simulink model "KitGewerk2_v14"  (R2014a)
settings: Solver=ode3  StartTime=0.0  StopTime=inf  FixedStep=0.005  RelTol=1e-3
undefined symbols (not defined in the file): Com1, Com2, none
libraries: slrtlib x14, dspswit3 x3, simulink x2, xpcseriallib x2
(part 2 of 2)

== matlab function KitGewerk2_v14/Robotino/serial communication/error filter & protocol disassembler ==
  settings: sampleTime=dtpc/2
  data: response input; error_free_resp_in input; direction_motor0_out output; velocity_motor0_out output; direction_motor1_out output; velocity_motor1_out output; direction_motor2_out output; velocity_motor2_out output; distance_measuring_sensors_out output; di03_bump_out output; bumper_out output; error_free_resp_out output
%%%%%%%%%%%%%%%%%%%%%%%%%%%%%%%%%%%%%%%%%%%%%%%%%%%%%%%%%%%%%%%%%%%%%%%%%%%
% Error check of the 'I/O-Board to PC104 message' and filtering of this   %
% defective response: Substitute defective message by the last error free %
% message.                                                                %
% Saving of the rotating direction, velocity, shaft position and running  %
% time of the three motors. Combining all shaft positions in a vector.    %
% Combining all running times in a vector.                                %
% Saving of the three bumper bytes indicating a collision in a vector.    %
% Saving the values of the nine distance measuring IR-sensors in a vector.%
%                                                                         %
% inputs: response (actual 'I/O-Board to PC104 message')(vector 102       %
%                   elements)                                             %
%         error_free_resp_in (last error free 'I/O-Board to PC104         %
%                             message')                                   %
% outputs: directions and velocities of the three motors                  %
%          motor_positions_out (shaft positions of the three motors)      %
%                              (vector 12 elements)                       %
%          time_bytes_out (running times of the three motors)             %
%                         (vector 9 elements)                             %
%          distance_measuring_sensors_out (values of the nine IR-sensors) %
%                                         (vector 9 elements)             %
%          bumper_out (vector 3 elements)                                 %
%          error_free_resp_out (error free 'I/O-Board to PC104 message')  %
%                              (vector 102 elements)                      %
%%%%%%%%%%%%%%%%%%%%%%%%%%%%%%%%%%%%%%%%%%%%%%%%%%%%%%%%%%%%%%%%%%%%%%%%%%%
function [direction_motor0_out, velocity_motor0_out, ...
          direction_motor1_out, velocity_motor1_out, ...
          direction_motor2_out, velocity_motor2_out, ...
          distance_measuring_sensors_out, di03_bump_out, bumper_out, ...
          error_free_resp_out] = fcn(response, error_free_resp_in)
%           motor_positions_out, time_bytes_out, ...)
      
%%%%%%%%%%%%%%%%%%%%%%%%%%%%%%%%%%%%%%%%%%%%%%%%%%%%%
% filtering defective 'I/O-Board to PC104 messages' %
%%%%%%%%%%%%%%%%%%%%%%%%%%%%%%%%%%%%%%%%%%%%%%%%%%%%%
if (response(1) == 101) && (response(2) == 82) && (response(3) == 69) ...
   && (response(4) == 67) && (response(100) == 114) ...        % if the ...
   && (response(101) == 101) && (response(102) == 99)  % counter (101), ...
                        % the start (REC) and stop (rec) bytes are true ...
    error_free_resp_out = response;     % save the actual 'I/O-Board to ...
                                                           % PC104 message'
else                                                        % otherwise ...
    error_free_resp_out = error_free_resp_in;     % save the last error ...
                                        % free 'I/O-Board to PC104 message'
end

%%%%%%%%%%%%%%%%%%%%%%%%%%%%%%%%%%%%%%%%%%%%%%%%%%%%%%%%%%%%%%%%%%%%%%%%%%
% save rotating direction, velocity, shaft position and the running time %
% of motor0                                                              %
%%%%%%%%%%%%%%%%%%%%%%%%%%%%%%%%%%%%%%%%%%%%%%%%%%%%%%%%%%%%%%%%%%%%%%%%%%
direction_motor0_out  = error_free_resp_out(26);
velocity_motor0_out   = error_free_resp_out(27);
% position_motor0_byte1 = error_free_resp_out(28);
% position_motor0_byte2 = error_free_resp_out(29);
% position_motor0_byte3 = error_free_resp_out(30);
% position_motor0_byte4 = error_free_resp_out(31);
% time_motor0_byte1     = error_free_resp_out(34);
% time_motor0_byte2     = error_free_resp_out(35);
% time_motor0_byte3     = error_free_resp_out(36);

%%%%%%%%%%%%%%%%%%%%%%%%%%%%%%%%%%%%%%%%%%%%%%%%%%%%%%%%%%%%%%%%%%%%%%%%%%
% save rotating direction, velocity, shaft position and the running time %
% of motor1                                                              %
%%%%%%%%%%%%%%%%%%%%%%%%%%%%%%%%%%%%%%%%%%%%%%%%%%%%%%%%%%%%%%%%%%%%%%%%%%
direction_motor1_out  = error_free_resp_out(47);
velocity_motor1_out   = error_free_resp_out(48);
% position_motor1_byte1 = error_free_resp_out(49);
% position_motor1_byte2 = error_free_resp_out(50);
% position_motor1_byte3 = error_free_resp_out(51);
% position_motor1_byte4 = error_free_resp_out(52);
% time_motor1_byte1     = error_free_resp_out(55);
% time_motor1_byte2     = error_free_resp_out(56);
% time_motor1_byte3     = error_free_resp_out(57);

%%%%%%%%%%%%%%%%%%%%%%%%%%%%%%%%%%%%%%%%%%%%%%%%%%%%%%%%%%%%%%%%%%%%%%%%%%
% save rotating direction, velocity, shaft position and the running time %
% of motor2                                                              %
%%%%%%%%%%%%%%%%%%%%%%%%%%%%%%%%%%%%%%%%%%%%%%%%%%%%%%%%%%%%%%%%%%%%%%%%%%
direction_motor2_out  = error_free_resp_out(68);
velocity_motor2_out   = error_free_resp_out(69);
% position_motor2_byte1 = error_free_resp_out(70);
% position_motor2_byte2 = error_free_resp_out(71);
% position_motor2_byte3 = error_free_resp_out(72);
% position_motor2_byte4 = error_free_resp_out(73);
% time_motor2_byte1     = error_free_resp_out(76);
% time_motor2_byte2     = error_free_resp_out(77);
% time_motor2_byte3     = error_free_resp_out(78);

%%%%%%%%%%%%%%%%%%%%%%%%%%%%%%%%%%%%%%%%%%%
% save the three bumper bytes in a vector %
%%%%%%%%%%%%%%%%%%%%%%%%%%%%%%%%%%%%%%%%%%%
bumper_out = [error_free_resp_out(32), error_free_resp_out(53), ...
              error_free_resp_out(74)]';
          
%%%%%%%%%%%%%%%%%%%%%%%%%%%%%%%%%%%%%%%%%%%%%%%%%%%%%%%%%%%%%%%%%%%%%%
% save the values of the nine distance measuring sensors in a vector %
%%%%%%%%%%%%%%%%%%%%%%%%%%%%%%%%%%%%%%%%%%%%%%%%%%%%%%%%%%%%%%%%%%%%%%
distance_measuring_sensors_out = [error_free_resp_out(60), ...
                    error_free_resp_out(59), error_free_resp_out(44), ...
                    error_free_resp_out(39), error_free_resp_out(38), ...
                    error_free_resp_out(17), error_free_resp_out(18), ...
                    error_free_resp_out(23), error_free_resp_out(65)];
                
%%%%%%%%%%%%%%%%%%%%%%%%%%%%%%%%%%%%%%%%%%%%%%%%%%%%%%%%
% save positions of the three motor shafts in a vector %
%%%%%%%%%%%%%%%%%%%%%%%%%%%%%%%%%%%%%%%%%%%%%%%%%%%%%%%%
% motor_positions_out = [position_motor0_byte1, position_motor0_byte2, ...
%                        position_motor0_byte3, position_motor0_byte4, ...
%                        position_motor1_byte1, position_motor1_byte2, ...
%                        position_motor1_byte3, position_motor1_byte4, ...
%                        position_motor2_byte1, position_motor2_byte2, ...
%                        position_motor2_byte3, position_motor2_byte4];

%%%%%%%%%%%%%%%%%%%%%%%%%%%%%%%%%%%%%%%%%%%%%%%%%%%%%%%%%%
% save the running times of the three motors in a vector %
%%%%%%%%%%%%%%%%%%%%%%%%%%%%%%%%%%%%%%%%%%%%%%%%%%%%%%%%%%
% time_bytes_out = [time_motor0_byte1, time_motor0_byte2, ...
%                   time_motor0_byte3, time_motor1_byte1, ...
%                   time_motor1_byte2, time_motor1_byte3, ...
%                   time_motor2_byte1, time_motor2_byte2, time_motor2_byte3];

%%%%%%%%%%%%%%%%%%%%%%%%%%%%%%%%%%%%%%
% save values of digital input 0 - 3 %
%%%%%%%%%%%%%%%%%%%%%%%%%%%%%%%%%%%%%%
di03_bump_out = error_free_resp_out(32);

== matlab function KitGewerk2_v14/Robotino/receive direction, unit & velocity converter ==
  settings: sampleTime=dtpc/2
  data: direction_motor0_in input; v_x_out output; velocity_motor0_in input; direction_motor1_in input; velocity_motor1_in input; direction_motor2_in input; velocity_motor2_in input; v_y_out output; v_theta_out output
%%%%%%%%%%%%%%%%%%%%%%%%%%%%%%%%%%%%%%%%%%%%%%%%%%%%%%%%%%%%%%%%%%%%%%%%%%%
% assembly of the three separate positive motor velocities (resolution:   %
% 1Byte) and their rotation direction to positive and/or negative         %
% longitudinal, lateral & rotational velocities (in milimeters per        %
% second)                                                                 %
%                                                                         %
% inputs:  direction_motor0_in (rotating direction of motor0              %
%          (129 := counter-clockwise; 128 := clockwise)),                 %
%          velocity_motor0_in (from 0 to 255),                            %
%          direction_motor1_in (rotating direction of motor1              %
%          (0 := counter-clockwise; 1 := clockwise)),                     %
%          velocity_motor1_in (from 0 to 255),                            %
%          direction_motor2_in (rotating direction of motor2              %
%          (0 := counter-clockwise; 1 := clockwise)),                     %
%          velocity_motor2_in (from 0 to 255)                             %
% outputs: v_x_out (longitudinal velocity (in milimeters per second)),    %
%          v_y_out (lateral velocity (in milimeters per second)),         %
%          v_theta_out (rotational velocity (in milimeters per second))   %
%%%%%%%%%%%%%%%%%%%%%%%%%%%%%%%%%%%%%%%%%%%%%%%%%%%%%%%%%%%%%%%%%%%%%%%%%%%
function [v_x_out, v_y_out, v_theta_out] ...
    = fcn(direction_motor0_in, velocity_motor0_in, direction_motor1_in, ...
          velocity_motor1_in, direction_motor2_in, velocity_motor2_in)
%%%%%%%%%%%%%%%%%%%%%%%%%%%%%%%%%%%%%%%%%%%%%%%%%%%%%%%%%%%%%%%%%
% assembly of absolute motor velocity and rotating direction to %
% longitudinal, lateral & rotational velocity for every motor   %
%%%%%%%%%%%%%%%%%%%%%%%%%%%%%%%%%%%%%%%%%%%%%%%%%%%%%%%%%%%%%%%%%
if direction_motor0_in < 129
    v0 = -velocity_motor0_in;
else
    v0 =  velocity_motor0_in;
end

if direction_motor1_in < 1
    v1 = -velocity_motor1_in;
else
    v1 =  velocity_motor1_in;
end

if direction_motor2_in < 1
    v2 = -velocity_motor2_in;
else
    v2 =  velocity_motor2_in;
end

%%%%%%%%%%%%%%%%%%%%%%%%%%%%%%%%%%%%%%%%%%%%%%%%%%%%%%%%%%%%%%%%%%%%%%%%%
% conversion of the separate motor velocities from a value between -255 %
% and 255 to millimeters                                                %
%%%%%%%%%%%%%%%%%%%%%%%%%%%%%%%%%%%%%%%%%%%%%%%%%%%%%%%%%%%%%%%%%%%%%%%%%
f_rcv = 7.02;
v0    = v0 * f_rcv;
v1    = v1 * f_rcv;
v2    = v2 * f_rcv;

%%%%%%%%%%%%%%%%%%%%%%%%%%%%%%%%%%%%%%%%%%%%%%%%%%%%%%%%%%%%%%%%%%%%
% conversion from three separate motor velocities to longitudinal, %
% lateral & rotational velocity                                    %
%%%%%%%%%%%%%%%%%%%%%%%%%%%%%%%%%%%%%%%%%%%%%%%%%%%%%%%%%%%%%%%%%%%%
v_x_out     = (v2 - v0) / (2 * cosd(30));                         % in mm/s
v_y_out     = (v0 - 2 * v1 + v2) / 3;                             % in mm/s
v_theta_out = (v0 + v1 + v2) / (3 * 135);                        % in rad/s

== matlab function KitGewerk2_v14/Begrenzung ==
  data: win input; wout output
function wout = fnc(win)
wert= zeros(1);
if win > 500
    wert = 500;
else
    wert = win;
end
wout = wert;

== matlab function KitGewerk2_v14/Robotino/serial communication/stop by bumper ==
  settings: sampleTime=2*dtpc
  data: stop_out output; bumper input; stop_flag_in input; stop_flag_out output
%%%%%%%%%%%%%%%%%%%%%%%%%%%%%%%%%%%%%%%%%%%%%%%%%%%%%%%%%%%%%%%%%%%%%%%%%%%
% Recognition of collisions and creating of variables indicating and      %
% marking a collision                                                     %
%                                                                         %
% inputs: bumper (vector of the three bumper bytes)                       %
%         stop_flag_in (As long as no collision has occured,              %
%                       'stop_flag_in' contains the last bumper vector    %
%                       indicating no collision.                          %
%                       If a collision has occured, 'stop_flag_in'        %
%                       contains the last bumper vector indicating a      %
%                       collision until the simulation stops.)            %
% outputs: stop_out (indicates a collision: 1 = no collision;             %
%                                           0 = collision)                %
%          stop_flag_out (gets the actual bumper vector unless 'bumper'   %
%                         indicates no collision and 'stop_flag_in'       %
%                         indicates a past collision.)                    %
%%%%%%%%%%%%%%%%%%%%%%%%%%%%%%%%%%%%%%%%%%%%%%%%%%%%%%%%%%%%%%%%%%%%%%%%%%%
function [stop_out, stop_flag_out] = fcn(bumper, stop_flag_in)
if max(bumper) == 31       % as soon as the maximum value of the bumper ...
                              % vector indicates 31 a collision is detected
    stop_out = 0;
    stop_flag_out = bumper;
elseif max(stop_flag_in) == 31 % if the maximum value of 'stop_flag_in' ...
                                      % indicates a past collision (31) ...
    stop_out = 0;         % 'stop_out' gets 0 for a further stop of the ...
                                                           % motors and ...
    stop_flag_out = stop_flag_in; % 'stop_flag_out' gets the last bumper...
                                       % vector indicating a past collision
else                                                        % otherwise ...
    stop_out = 1;    % 'stop_out' gets 1 to keep the motors running and ...
    stop_flag_out = bumper; % 'stop_flag_out' gets the actual bumper vector
end

== matlab function KitGewerk2_v14/Robotino/distance converter ==
  settings: sampleTime=dtpc/2
  data: dms_in input; dms_out output
%%%%%%%%%%%%%%%%%%%%%%%%%%%%%%%%%%%%%%%%%%%%%%%%%%%%%%%%%%%%%%%%%%%%%%%%%%%
% conversion of the nine distance measuring sensor values (resolution:    %
% 1Byte) to unit milimeters (range: from 40mm to 1500mm) with linear      %
% interpolation                                                           %
%                                                                         %
% input:  vector containing the values of the nine distance measuring     %
%         sensors                                                         %
% output: vector containing the nine values in milimeters                 %
%%%%%%%%%%%%%%%%%%%%%%%%%%%%%%%%%%%%%%%%%%%%%%%%%%%%%%%%%%%%%%%%%%%%%%%%%%%
function dms_out = fcn(dms_in)

y_mm = [40, 45, 50, 60, 75, 100, 125, 150, 175, 200, 250, 300]; % , ...
        %400, 500, 600, 700, 800, 900, 1000, 1100, 1200, 1300, 1500];
    
x_sensor = [255, 249.7733813, 228.6082474, 193.6871795, ...
            152.0044843, 113.7266187, 92.42268041, ...
            76.36407767, 65.19289827, 55.1025641, ...
            43.06299213, 34.97068404]; % , 24.37410072, ...
            % 16.3381295, 11.62589928, 8.661870504, ...
            % 6.316546763, 4.74, 3.65, 2.96, 2.40, ...
            % 2.035971223, 1.539568345];

% x_sensor = round(100 * x_sensor) / 100;

dms_out = interp1(x_sensor, y_mm, dms_in, 'linear');

== matlab function KitGewerk2_v14/Robotino/assemble robotino response ==
  data: v_x_in input; robotino_response output; v_y_in input; v_theta_in input; distance_measuring_sensors_in input; bumper_in input; light_barrier_in input; slider_in input
%%%%%%%%%%%%%%%%%%%%%%%%%%%%%%%%%%%%%%%%%%%%%%%%%%%%%%%%%%%%%%%%%%%%%%%%%%%
% Assembly of robot data in a vector of 34 elements.                      %
%                                                                         %
% inputs:   longitudinal, lateral and rotational velocity (in mm/s),      %
%           shaft positions of the three motors (4 elements per motor),   %
%           running times of the three motors (3 elements per motor),     %
%           values of the nine IR-sensors (in mm),                        %
%           bumper collision (1 = no collision;                           %
%                             0 = collision)                              %
% outputs:  vector containing assembled input data                        %
%%%%%%%%%%%%%%%%%%%%%%%%%%%%%%%%%%%%%%%%%%%%%%%%%%%%%%%%%%%%%%%%%%%%%%%%%%%
function robotino_response = fcn(v_x_in, v_y_in, v_theta_in, ...
                                 distance_measuring_sensors_in, ...
                                 bumper_in, light_barrier_in, slider_in)
                                 % motor_positions_in, time_bytes_in, ...)
robotino_response = [light_barrier_in, slider_in, v_x_in, v_y_in, ...
                     v_theta_in, ...%motor_positions_in, time_bytes_in, ...
                     distance_measuring_sensors_in, bumper_in]';

== matlab function KitGewerk2_v14/Robotino/light barrier & slider ==
  data: di03_bump_in input; light_barrier output; slider output
function [light_barrier, slider] = fcn(di03_bump_in)
%%%%%%%%%%%%%%%%%%%%%%%%%%%%%%%%%%%%%%%%%%%%%%%%%%%%%%%%%%%%%%%%%%%%%%%%%%%
% di03_bump_in = 0 alternatively 12 ->  no light barrier activation       %
%                                       no slider activation              %
% di03_bump_in = 13                 ->  only light barrier activation     %
% di03_bump_in = 14                 ->  only slider activation            %
% di03_bump_in = 15                 ->  light barrier activation          %
%                                       slider activation                 %
%%%%%%%%%%%%%%%%%%%%%%%%%%%%%%%%%%%%%%%%%%%%%%%%%%%%%%%%%%%%%%%%%%%%%%%%%%%
% function [light_barrier, slider] = fcn(di03_bump_in)
% bin = dec2bin(di03_bump_in);
% if bin(3) == 1
%     light_barrier = 1;
% else
%     light_barrier = 0;
% end
% if bin(4) == 1
%     slider = 1;
% else
%     slider = 0;
% end
if     di03_bump_in == 13
    light_barrier = 1;
    slider        = 0;
elseif di03_bump_in == 14
    light_barrier = 0;
    slider        = 1;
elseif di03_bump_in == 15
    light_barrier = 1;
    slider        = 1;
else
    light_barrier = 0;
    slider        = 0;
end

== matlab function KitGewerk2_v14/Begrenzung1 ==
  data: win input; wout output
function wout = fnc(win)
wert= zeros(1);
if win > 500
    wert = 500;
else
    wert = win;
end
wout = wert;

== matlab function KitGewerk2_v14/Begrenzung2 ==
  data: win input; wout output
function wout = fnc(win)
wert= zeros(1);
if win > 3,14
    wert = 3,14;
else
    wert = win;
end
wout = wert;

== matlab function KitGewerk2_v14/Gewerk_2/Kollisionserkennung ==
  data: d_Abstand input; b_stop output boolean; ad_Abstandssensor input
function b_stop = fcn(d_Abstand,ad_Abstandssensor)
b_stop=false;
if sum(isnan(ad_Abstandssensor))==9 % nan = kein Hinderniss
    % kein Hinderniss   
    b_stop= false; 
else
    % Hinderniss entdeckt, min. ein Sensor(kein nan)
    if ( (ad_Abstandssensor(1)<d_Abstand) || (ad_Abstandssensor(2)<d_Abstand) || (ad_Abstandssensor(3)<d_Abstand) || ...
         (ad_Abstandssensor(4)<d_Abstand) ||(ad_Abstandssensor(5)<d_Abstand) ||(ad_Abstandssensor(6)<d_Abstand) || ...
         (ad_Abstandssensor(7)<d_Abstand) || (ad_Abstandssensor(8)<d_Abstand) ||(ad_Abstandssensor(9)<d_Abstand)) 

    b_stop= true;
    end
end

== matlab function KitGewerk2_v14/Gewerk_2/MATLAB Function ==
  data: ad_PL input; d_Y_soll output double; d_X_soll output double; d_Phi_soll output double; d_V_Max_soll output double; int_I input
function [d_Y_soll,d_X_soll,d_Phi_soll,d_V_Max_soll]= fcn(ad_PL,int_I)

int_I=int_I+1; %Offset, da Zeilenindex bei 1 beginnt



if (ad_PL(int_I,1)<0 || ad_PL(int_I,2)<0 || ad_PL(int_I,3)<0 || ad_PL(int_I,4)<0)
int_I = int_I-1;
end 

d_Y_soll= ad_PL(int_I,1);
d_X_soll= ad_PL(int_I,2);
d_Phi_soll= ad_PL(int_I,3);
d_V_Max_soll= ad_PL(int_I,4);

== stateflow chart KitGewerk2_v14/Gewerk_2/Chart ==
  state Routinen_Stationen
    state Wegpunktliste_erstellen_state
      entry: A_WPL=Wegpunktliste_erstellen(UI_Auftrnr,uint8(B_Endst))
      B_WPL_cnt_reset =true
    state Werkstueck_aufnehmen
      state Fahrt_zu_Platz1
        entry: B_WPL_cnt_reset=false
      state Greifer_schließen
        entry:B_WP_weiter=true
        B_Greifer= true
        B_Stop=true
        exit:B_Stop=false
      state Weiterfahren_zu_RFID
        entry:B_WP_weiter=false
      state RFID_lesen_2
        during: UI_to_GW1= uint8(2)
        B_Stop=true
        exit:B_Stop=false
        B_WP_weiter=true
      state WP_weiterschalten_3
      state Routine_fertig
        entry: B_Endst=true
      Fahrt_zu_Platz1 -> Greifer_schließen : [B_Schieber&&B_Lichtschranke]
      Greifer_schließen -> Weiterfahren_zu_RFID : after(500,msec)
      Weiterfahren_zu_RFID -> RFID_lesen_2 : [B_Schieber]
      RFID_lesen_2 -> WP_weiterschalten_3 : [UI_from_GW1==2]
      WP_weiterschalten_3 -> Routine_fertig : /{B_WP_weiter=false}
    state Werkstueck_ablegen
      state Fahrt_zu_RFID
        entry: B_WPL_cnt_reset=false
      state RFID_lesen
        entry: UI_to_GW1= uint8(4)
        B_Stop=true
        exit:B_Stop=false
        B_WP_weiter=true
      state WP_weiterschalten
      state Fahrt_zu_Ablage
        entry: B_WP_weiter=false
      state Greifer_Oeffnen
        entry: B_Stop=true
        B_Greifer=false
        B_WP_weiter=true
      state WP_weiterschalten2
        entry:
        B_Stop=false
      state Auftrag_fertig
        entry: B_WP_weiter=false
        exit:UI_to_GW1= uint8(5)
        B_Endst=false
      Fahrt_zu_RFID -> RFID_lesen : [B_Schieber]
      RFID_lesen -> WP_weiterschalten : [UI_from_GW1==4]
      WP_weiterschalten -> Fahrt_zu_Ablage
      Fahrt_zu_Ablage -> Greifer_Oeffnen : [B_Schieber]
      Greifer_Oeffnen -> WP_weiterschalten2 : after(500,msec)
      WP_weiterschalten2 -> Auftrag_fertig
    (default) -> Wegpunktliste_erstellen_state
    Wegpunktliste_erstellen_state -> Fahrt_zu_RFID [order 1] : [B_Endst==true]
    Wegpunktliste_erstellen_state -> Fahrt_zu_Platz1 [order 2] : [B_Endst==false]
  state Station_aendern
    entry: if B_Endst==false
    UI_Auftrnr=UI_Startstation
    else
    UI_Auftrnr=UI_Endstation
    end
  state Fahrt_in_nav_2
  state Nav2_abfrage
  state Eintrittspunkt_erreicht
  state A_stern_fahrt
    state A_stern
    state Kollisionserkennung
      entry:
      if B_Endst==false
      UI_to_GW1=uint8(1) %Startplatz für GW1 freigeben
      else
      UI_to_GW1=uint8(3) %Endplatz für GW1 freigeben
      end
    A_stern -> Kollisionserkennung : [WP_cnt>1]
        | % Sobald der Zähler>1
        | % befindet sich der
        | % Robi im Feld
    (default) -> A_stern
  state Stationsentscheider
    entry: if B_Endst==false
    UI_Auftrnr=UI_Startstation
    else
    UI_Auftrnr=UI_Endstation
    end
  state Fahrt_zum_Warteplatz
    entry:A_stern_test=simfcn()
    state Out1 = simfcn [function]
  state Auftrag_empfangen
    exit:
    UI_Startstation=UI_Startstation_in
    UI_Endstation=UI_Endstation_in
    %Eingänge speichern
  state Init
    entry: B_Endst=false
  state Warten_auf_Auftrag
  state Warten_auf_neuen_Auftrag
  state Routinen_Warteplaetze
  state Routinen_Ladestationen
    state Warten_auf_Ereignis
    state Laden_beenden
    state Laden_beginnen
    state Fahrt_an_rand_nav1
    state Wegpunkte
    state Kontakt_fehler
    Laden_beenden -> Fahrt_an_rand_nav1
    Wegpunkte -> Laden_beginnen : [B_last_WP && B_da]
    Laden_beginnen -> Warten_auf_Ereignis [order 2]
    (default) -> Wegpunkte
    Warten_auf_Ereignis -> Laden_beenden
    Kontakt_fehler -> Laden_beginnen : [B_last_WP && B_da]
    Laden_beginnen -> Kontakt_fehler [order 1]
  state Auftrag_empfangen1
    exit:
    UI_Startstation=UI_Startstation_in
    UI_Endstation=UI_Endstation_in
    %Eingänge speichern
  Kollisionserkennung -> Eintrittspunkt_erreicht : [B_last_WP && B_da ...
      | &&( UI_from_GW1==1 || UI_from_GW1==3)]
  Nav2_abfrage -> A_stern_fahrt [order 1]
  Fahrt_an_rand_nav1 -> Stationsentscheider : [B_last_WP && B_da]
  Station_aendern -> Routinen_Stationen
  Fahrt_in_nav_2 -> Station_aendern
  Eintrittspunkt_erreicht -> Routinen_Stationen [order 1] : [UI_Auftrnr<=16]
  Nav2_abfrage -> Fahrt_in_nav_2 [order 2]
  Warten_auf_Auftrag -> Auftrag_empfangen : [UI_Startstation_in==200 ...
      | && UI_Endstation_in==200]...
      |  /{UI_to_GW1= uint8(200)}
  Auftrag_empfangen -> Stationsentscheider : [UI_Startstation_in<200 ...
      | && UI_Endstation_in<200]
  Fahrt_zum_Warteplatz -> Warten_auf_Auftrag : [B_last_WP && B_da]
  Init -> Fahrt_zum_Warteplatz
  Eintrittspunkt_erreicht -> Routinen_Warteplaetze [order 2] : [UI_Auftrnr>16 &&  UI_Auftrnr<=20]
  Stationsentscheider -> A_stern_fahrt
  (default) -> Init
  Routinen_Warteplaetze -> Warten_auf_neuen_Auftrag
  Warten_auf_neuen_Auftrag -> Auftrag_empfangen1 : [UI_Startstation_in==200&& UI_Endstation_in==200]...
      |  /{UI_to_GW1= uint8(200)}
  Eintrittspunkt_erreicht -> Routinen_Ladestationen [order 3] : [UI_Auftrnr>20]
  Auftrag_empfangen1 -> Stationsentscheider : [UI_Startstation_in<200 ...
      | && UI_Endstation_in<200]
  Routine_fertig -> Nav2_abfrage
  Auftrag_fertig -> Warten_auf_neuen_Auftrag : [B_last_WP && B_da]
  data: Auftragsnummer function_input; Is_Endstation function_input; Wegpunktliste function_output; Out1 function_output; Auftragsnummer function_input; Wegpunktliste function_output; B_Endst local boolean; UI_Auftrnr local uint8 size=1; A_WPL output; B_Schieber input boolean size=1; UI_from_GW1 input uint8 size=1; B_Stop output boolean size=1; B_WP_weiter output boolean size=1; B_Greifer output boolean size=1; B_Lichtschranke input boolean size=1; B_WPL_cnt_reset output boolean size=1; UI_to_GW1 output uint8 size=1; B_last_WP input boolean size=1; UI_Startstation local uint8 size=1; UI_Endstation local uint8 size=1; B_da input boolean size=1; UI_Robi_ID input uint8 size=1; WP_cnt input size=1; UI_Endstation_in input uint8 size=1; UI_Startstation_in input uint8 size=1; A_stern_test output
  function Wegpunktliste= Wegpunktliste_erstellen(Auftragsnummer,Is_Endstation):
    | function Wegpunktliste= Wegpunktliste_erstellen(Auftragsnummer,Is_Endstation) 
    | 
    | Wegpunktliste=zeros(50,4); %Intitialisierung WPL mit 50 Elementen
    | Wegpunktliste(:,:)=-1;
    | 
    | switch Auftragsnummer  
    | 
    |     case {2 , 1}
    |     offset_Station=0;    %Offset in X-Richtung
    |     links_rechts=0;      %0= links , 1= vorne
    |     case {3 , 4}
    |     offset_Station=0;
    |     links_rechts=1;
    |     case {5 , 6}
    |     offset_Station=1200;
    |     links_rechts=0;
    |     case {7 , 8}
    |     offset_Station=1200;
    |     links_rechts=1;
    |     case {9 , 10}
    |     offset_Station=2400;
    |     links_rechts=0;
    |     case {11 , 12}
    |     offset_Station=2400;
    |     links_rechts=1;
    |     case {13 , 14}
    |     offset_Station=3600;
    |     links_rechts=0;
    |     case {15 , 16}
    |     offset_Station=3600;
    |     links_rechts=1;
    |     otherwise
    |     offset_Station=-1000;    
    |     links_rechts=0;  
    |     
    | end
    | 
    | 
    | %platz vorne(stirnseite)=1, hinten (Platz nähe RFID)=0
    | hinten_vorne = mod(Auftragsnummer,2); 
    | 
    | 
    | 
    | 
    | %***** Statische Listen *****
    | %Bezogen auf die Erste Station (Rohteillager)
    | 
    | %Koordinaten für Plätze
    | %Alle Plätze müssen die gleich Länge haben
    | Platz_1=[1 1 1 1;11 11 11 11;111 111 111 111];
    | Platz_2=[2 2 2 2;22 22 22 22;222 222 222 222];
    | Platz_3=[3 3 3 3;33 33 33 33;333 333 333 333];
    | Platz_4=[4 4 4 4;44 44 44 44;444 444 444 444];
    | RFID_L=[5 5 5 5;55 55 55 55;555 555 555 555];
    | RFID_R=[6 6 6 6;66 66 66 66;666 666 666 666];
    | 
    | Anz_WP=3; %Anzahl Wegpunkt (gleiche Anzahl für alle Plätze)
    | 
    | 
    | 
    | %**** Auswahl der Richtigen Wegpunktliste *****
    | 
    |  
    | 
    | % **** Ablegen ****
    | if links_rechts==0 && Is_Endstation==1 %Werkstück ablegen linke Seite
    |     
    |     Wegpunktliste(1:Anz_WP,1:4)=RFID_L;
    |    
    |     if hinten_vorne == 1 %Wegpunkte für Platz 1 zuweisen
    |         Wegpunktliste((Anz_WP+1):(2*Anz_WP),1:4)=Platz_1;
    |     end
    |     
    |     if hinten_vorne == 0 % Wegpunkte für Platz 2 zuweisen
    |         Wegpunktliste((Anz_WP+1):(2*Anz_WP),1:4)=Platz_2;
    |     end
    |     
    |    
    | end
    | 
    | 
    | if links_rechts==1 && Is_Endstation==1 %Werkstück ablegen rechte Seite
    |        
    |         Wegpunktliste(1:Anz_WP,1:4)=RFID_R;
    |    
    |     if hinten_vorne == 1 %Wegpunkte für Platz 1 zuweisen
    |         Wegpunktliste((Anz_WP+1):(2*Anz_WP),1:4)=Platz_3;
    |     end
    |     
    |     if hinten_vorne == 0 % Wegpunkte für Platz 2 zuweisen
    |         Wegpunktliste((Anz_WP+1):(2*Anz_WP),1:4)=Platz_4;
    |     end
    |    
    |     
    | end
    |     
    | %****Werkstück aufnehmen*****   
    |     
    | if links_rechts==0 && Is_Endstation==0 %Werkstück ablegen linke Seite
    |     
    |    
    |     if hinten_vorne == 1 %Wegpunkte für Platz 1 zuweisen
    |         Wegpunktliste(1:Anz_WP,1:4)=Platz_1;
    |     end
    |     
    |     if hinten_vorne == 0 % Wegpunkte für Platz 2 zuweisen
    |         Wegpunktliste(1:Anz_WP,1:4)=Platz_2;
    |     end
    |     
    |     
    |     
    |     Wegpunktliste((Anz_WP+1):(2*Anz_WP),1:4)=RFID_L;
    | end
    | 
    | 
    | if links_rechts==1 && Is_Endstation==0 %Werkstück ablegen linke Seite
    |     
    |    
    |     if hinten_vorne == 1 %Wegpunkte für Platz 1 zuweisen
    |         Wegpunktliste(1:Anz_WP,1:4)=Platz_3;
    |     end
    |     
    |     if hinten_vorne == 0 % Wegpunkte für Platz 2 zuweisen
    |         Wegpunktliste(1:Anz_WP,1:4)=Platz_4;
    |     end
    |   
    |     
    |     
    |     Wegpunktliste((Anz_WP+1):(2*Anz_WP),1:4)=RFID_R;
    | end
    | 
    | 
    | %X Werte um Offset erhöhen
    | 
    | Wegpunktliste(1:(2*Anz_WP),:)=[Wegpunktliste(1:(2*Anz_WP),1)+offset_Station Wegpunktliste(1:(2*Anz_WP),2:4)]
    | 
    | end
  function Wegpunktliste= Wegpunktliste_Wartepl(Auftragsnummer):
    | function Wegpunktliste= Wegpunktliste_Wartepl(Auftragsnummer)
    | 
    | Wegpunktliste=zeros(50,4); %Intitialisierung WPL mit 50 Elementen
    | Wegpunktliste(:,:)=-1;
    | switch Auftragsnummer 
    |     
    |     case 17
    |     
    |     case 18
    |     case 19
    |     case 20
    |     otherwise
    |     
    | end
    | 
    | 
    | 
    | end

== matlab function KitGewerk2_v14/Power Management Gewerk 4/Output_Flag-Comparison: Blei oder Li-ION ==
  data: Output_Flag_Li_Io input; Output_Flag_Blei input; Output_Flag output; Rob_ID input
function Output_Flag = ifid(Output_Flag_Li_Io, Output_Flag_Blei, Rob_ID)

if (Rob_ID == 4 || Rob_ID == 3)
    Output_Flag = Output_Flag_Li_Io;
else
    Output_Flag = Output_Flag_Blei;
end

== matlab function KitGewerk2_v14/Power Management Gewerk 4/Robotiono 1 and 2: Simulation of Charging and Discharging/Simulation of Charging and Discharging/Flag Communication Simulation ==
  data: Input_Flag input; Output_Flag output
function Output_Flag = Flag_Simulation(Input_Flag)

if Input_Flag == 1
    Output_Flag = 1;

elseif Input_Flag == 2
    Output_Flag = 2;

else
    Output_Flag = 0;
end


end

== matlab function KitGewerk2_v14/Power Management Gewerk 4/Robotiono 1 and 2: Simulation of Charging and Discharging/Simulation of Charging and Discharging/MATLAB Function ==
  data: Cnt input uint16; Inc input double; y output double
function y = fcn(Cnt, Inc)

if Cnt >= 3000
    y = 0;
else
    y = double(Inc);
end

== matlab function KitGewerk2_v14/Power Management Gewerk 4/Robotiono 1 and 2: Simulation of Charging and Discharging/Simulation of Charging and Discharging/MATLAB Function1 ==
  data: Cnt input uint32; Inc input uint8; y output double
function y = fcn(Cnt, Inc)

if Cnt <= 2
    y = 0;
else
    y = double(Inc);
end

== matlab function KitGewerk2_v14/Power Management Gewerk 4/Robotiono 3 and 4: Communication with Feature Pack 4.0/Microcontroller Data ==
  settings: sampleTime=dtpc/2
  data: Received_Data input; SOC output; FLAG output; Previous_Flag input; Previous_SOC input

%%%%%%%%%%%%%%%%%%%%%%%%%%%%%%%%%%%%%%%%%%%%%%%%%%%%%%%%%%%%%%%%%%%%%%%%%%%
% Error check of the 'I/O-Board to PC104 message' and filtering of this   %
% defective response: Substitute defective message by the last error free %
% message.                                                                %
% Saving of the rotating direction, velocity, shaft position and running  %
% time of the three motors. Combining all shaft positions in a vector.    %
% Combining all running times in a vector.                                %
% Saving of the three bumper bytes indicating a collision in a vector.    %
% Saving the values of the nine distance measuring IR-sensors in a vector.%
%                                                                         %
% inputs: response (actual 'I/O-Board to PC104 message')(vector 102       %
%                   elements)                                             %
%         error_free_resp_in (last error free 'I/O-Board to PC104         %
%                             message')                                   %
% outputs: directions and velocities of the three motors                  %
%          motor_positions_out (shaft positions of the three motors)      %
%                              (vector 12 elements)                       %
%          time_bytes_out (running times of the three motors)             %
%                         (vector 9 elements)                             %
%          distance_measuring_sensors_out (values of the nine IR-sensors) %
%                                         (vector 9 elements)             %
%          bumper_out (vector 3 elements)                                 %
%          error_free_resp_out (error free 'I/O-Board to PC104 message')  %
%                              (vector 102 elements)                      %
%%%%%%%%%%%%%%%%%%%%%%%%%%%%%%%%%%%%%%%%%%%%%%%%%%%%%%%%%%%%%%%%%%%%%%%%%%%
function [SOC, FLAG] = fcn(Received_Data, Previous_Flag, Previous_SOC)

FLAG = Received_Data(3);
SOC = Received_Data(2);



if (SOC > 106 || SOC < 0)
    SOC = Previous_SOC;
end

if (FLAG > 6 || FLAG < 0)
    FLAG = Previous_Flag;
end




%           motor_positions_out, time_bytes_out, ...)

== matlab function KitGewerk2_v14/Power Management Gewerk 4/SOC-Comparison: Blei oder Li-ION ==
  data: LiIO_SOC input; Blei_SOC input; Output_SOC output; Rob_ID input
function Output_SOC = ifid(LiIO_SOC, Blei_SOC, Rob_ID)

if (Rob_ID == 4 || Rob_ID == 3)
    Output_SOC = LiIO_SOC;
else
    Output_SOC = Blei_SOC;
end

== matlab function KitGewerk2_v14/Power Management Gewerk 4/Robotiono 1 and 2: Simulation of Charging and Discharging/Simulation of Charging and Discharging/Unterscheidung Blei Gel Roboter an der virtuellen Ladestation ==
  data: Input_Flag input; Laden output
 function Laden = fcn(Input_Flag)

 if (Input_Flag == 1)  
     
    Laden=1;  
    
 else
     
    Laden=0;    
    
 end
 
 
 
 end

== matlab function KitGewerk2_v14/Power Management Gewerk 4/Robotiono 1 and 2: Simulation of Charging and Discharging/Simulation of Charging and Discharging/Relais ansteuern1 ==
  data: Laden input; SOC1 input; SOC2 input; SOC output
function SOC = fcn(Laden, SOC1, SOC2)

if Laden == 1 
    SOC = SOC1;
else    
    SOC = SOC2;
end
